simulink library "Dampers_Axle1_Interconnected"  (R2025b)
settings: Solver=VariableStepAuto  StartTime=0.0  StopTime=10.0  RelTol=1e-3
libraries: Damper_LeftRight x1
Description:
  | Component of Simscape Vehicle Templates Library
  | 
  | Copyright 2018-2025 The MathWorks, Inc.
settings Model: Creator=smiller  LastModifiedBy=smiller
settings SolverCC: AlgebraicLoopSolver=TrustRegion
settings DataIOCC: ReturnWorkspaceOutputs=off
settings OptimizationCC: ReuseModelBlockBuffer=off
settings DebuggingCC: UnconnectedInputMsg=warning  UnconnectedOutputMsg=warning  UnconnectedLineMsg=warning  ArithmeticOperatorsInVariantConditions=warning
settings ModelReferenceCC: EnableRefExpFcnMdlSchedulingChecks=on
settings SFSimCC: CustomCodeUndefinedFunction=UseInterfaceOnly
settings RTWCC: GPUComputeCapability=3.5  DLArmComputeVersion=19.05

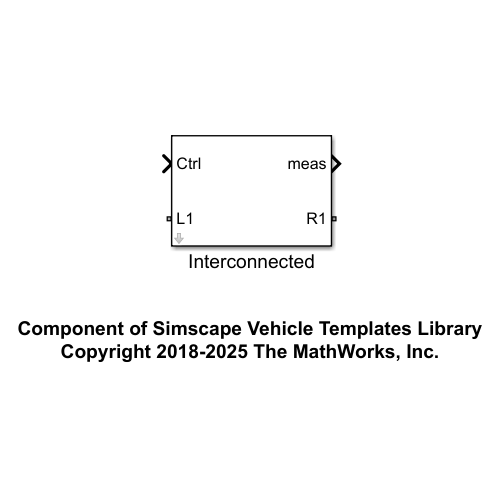
[thumbnail: Simulink's stored preview of the top-level diagram]
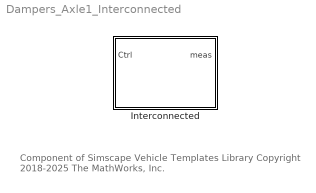
== system Dampers_Axle1_Interconnected ==
  note: Component of Simscape Vehicle Templates Library
      | Copyright 2018-2025 The MathWorks, Inc.
  Interconnected : Subsystem  VariantControl=Interconnected  mask(Interconnected Dampers){}
      mask help: Dampers connected across an axle.

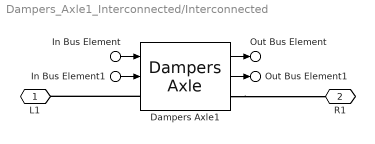
== system Dampers_Axle1_Interconnected/Interconnected ==
  In Bus Element1 : Inport  PortName=Ctrl  Element=R1
  In Bus Element : Inport  PortName=Ctrl  Element=L1
  Dampers Axle1 : Damper_LeftRight/Dampers Axle  VariantControl=Variant1  LabelModeActiveChoice=Linear  Damper=Damper.Axle1  VariantLabel=Damper.Axle1.class.Value
      settings: AttributesFormatString=%<ActiveVariant>
  L1 : PMIOPort  Side=Left
  R1 : PMIOPort  Port=2  Side=Right
  Out Bus Element : Outport  VectorParamsAs1DForOutWhenUnconnected=off  PortName=meas  Element=L1
  Out Bus Element1 : Outport  VectorParamsAs1DForOutWhenUnconnected=off  PortName=meas  Element=R1
  wires:
  In Bus Element/1 -> Dampers Axle1/1
  In Bus Element1/1 -> Dampers Axle1/2
  Dampers Axle1/1 -> Out Bus Element/1
  Dampers Axle1/2 -> Out Bus Element1/1
  connections:
  Dampers Axle1/LConn1 -- L1/RConn1
  Dampers Axle1/RConn1 -- R1/RConn1
